simulink model "EvPowertrainController4EM"  (R2026b)
model workspace (MAT data in the model file):
  CtrlVcuAccelPdlBpts = [0 0.8 1]
  CtrlVcuBattPnlty = 10000000
  CtrlVcuBattSOCBpts = [0 20 60 80 100]
  CtrlVcuCnstrntPnltyFctr = 10000000
  CtrlVcuEMPnlty = 100
  CtrlVcuEMTrqSplitGrid = 200
  CtrlVcuFallRate = -500
  CtrlVcuMaxAccelG = 1
  CtrlVcuMaxDecelG = -1.5
  CtrlVcuPwrDeltaPnlty = 50
  CtrlVcuPwrRatePnlty = [25 25 100]
  CtrlVcuRiseRate = 500
  CtrlVcuRoadMuEst = 0.8
  CtrlVcuSftyFctr = 0.9
  CtrlVcuTracPwrErrPnlty = 25
  CtrlVcuTrqVecBrkThresh = 0.01
  CtrlVcuTrqVecIGain = 0
  CtrlVcuTrqVecMinTrq = 25
  CtrlVcuTrqVecPGain = -2000
  CtrlVcuTrqVecSteerThresh = 0.349065850399
  CtrlVcuTrqVecVelThresh = 2.5
  N_P0 = 3
undefined symbols (not defined in the file): CtrlBcuTrlrBrkGain, CtrlVcuEvChrgLmtBpt, CtrlVcuEvRegenBrkCutOff, CtrlVcuEvRegenBrkSpdBpt, CtrlVcuEvSocBpt, eff, EnvGrvty, PlntBrkActrBoreFrnt, PlntBrkActrBoreRear, PlntBrkFrntBias, PlntBrkKinFricCffFrnt, PlntBrkKinFricCffRear, PlntBrkNumPadsFrnt, PlntBrkNumPadsRear, PlntBrkPadMeanRadiusFrnt, PlntBrkPadMeanRadiusRear, PlntBrkPrsFctr, PlntBrkRearBias, PlntDiffrntl2Eff, PlntDiffrntl2Ratio, PlntDiffrntlEff, PlntDiffrntlRatio, PlntEM1EffTbl, PlntEM1Spd, PlntEM1SpdEff, PlntEM1TransEff, PlntEM1TransGearRatio, PlntEM1Trq, PlntEM1TrqEff, PlntEM2EffTbl, PlntEM2Spd, PlntEM2SpdEff, PlntEM2TransEff, PlntEM2TransGearRatio, PlntEM2Trq, PlntEM2TrqEff, PlntEM3EffTbl, PlntEM3Spd, PlntEM3SpdEff, PlntEM3TransEff, PlntEM3TransGearRatio, PlntEM3Trq, PlntEM3TrqEff, PlntEMWhlGearEffFL, PlntEMWhlGearEffRL, PlntEMWhlGearRatioFL, PlntEMWhlGearRatioRL, PlntTransEffSpdBpt, PlntTransEffTbl, PlntTransEffTempBpt, PlntTransEffTrqBpt, PlntTransGearNumVect, PlntTransGearRatioVect, PlntVehCGHgtAxl, PlntVehDstCGFrntAxl, PlntVehDstCGRearAxl, PlntVehMass, PlntWhlLdRadiusFrnt, PlntWhlLdRadiusRear
libraries: simulink x11, sl_discontinuities x6, autolibutils x2, slpidlib x2
(part 5 of 5)

== system EvPowertrainController4EM/Energy Management/Calculate Average EMSpd and Wheel Torque Curves for Front and Rear Axles/3EM Dual Front/EMTrq2WhlTrqFrnt/Single Speed Transmission/Gear Eta ==
  note: Pwr >= 0, v = 1
      | Pwr < 0, v= -1
  SpdIn : Inport
  TrqIn : Inport  Port=2
  Constant : Constant  Value=PlntEMWhlGearEffFL*PlntEM1TransEff
  Constant1 : Constant  SampleTime=-1
  Constant2 : Constant  Value=-1  SampleTime=-1
  Math Function1 : Math  Operator=pow  SignedPower=on  OutputSignalType=real
  Product1 : Product
  Switch2 : Switch  SaturateOnIntegerOverflow=off  InputSameDT=off
  eta : Outport  VectorParamsAs1DForOutWhenUnconnected=off
  wires:
  TrqIn/1 -> Product1/1
  Math Function1/1 -> eta/1
  Switch2/1 -> Math Function1/2
  Product1/1 -> Switch2/2
  Constant1/1 -> Switch2/1
  Constant2/1 -> Switch2/3
  Constant/1 -> Math Function1/1
  SpdIn/1 -> Product1/2

== system EvPowertrainController4EM/Energy Management/Calculate Average EMSpd and Wheel Torque Curves for Front and Rear Axles/3EM Dual Front/EMTrq2WhlTrqFrnt/Transmission/Diff Eta ==
  SpdIn : Inport
  TrqIn : Inport  Port=2
  Constant : Constant  Value=PlntDiffrntlEff
  Constant1 : Constant  SampleTime=-1
  Constant2 : Constant  Value=-1  SampleTime=-1
  Math Function1 : Math  Operator=pow  SignedPower=on  OutputSignalType=real
  Product1 : Product
  Switch2 : Switch  SaturateOnIntegerOverflow=off  InputSameDT=off
  eta : Outport  VectorParamsAs1DForOutWhenUnconnected=off
  wires:
  TrqIn/1 -> Product1/1
  Math Function1/1 -> eta/1
  Switch2/1 -> Math Function1/2
  Product1/1 -> Switch2/2
  Constant1/1 -> Switch2/1
  Constant2/1 -> Switch2/3
  Constant/1 -> Math Function1/1
  SpdIn/1 -> Product1/2

== system EvPowertrainController4EM/Energy Management/Calculate Average EMSpd and Wheel Torque Curves for Front and Rear Axles/3EM Dual Front/EMTrq2WhlTrqFrnt/Transmission/Trans Eta ==
  TrqIn : Inport
  SpdIn : Inport  Port=2
  Gear : Inport  Port=3
  Abs1 : Abs  SaturateOnIntegerOverflow=off
  Constant : Constant  Value=PlntTransEffTempBpt(1)
  Constant1 : Constant  SampleTime=-1
  Constant2 : Constant  Value=-1  SampleTime=-1
  Eta 4D : Lookup_n-D  NumberOfTableDimensions=4  LookupTableObject=''  BreakpointsForDimension1=PlntTransEffTrqBpt  BreakpointsForDimension2=PlntTransEffSpdBpt  BreakpointsForDimension3=PlntTransGearNumVect  BreakpointsForDimension4=PlntTransEffTempBpt  Table=PlntTransEffTbl  ExtrapMethod=Clip  InternalRulePriority=Speed  RndMeth=Simplest
      settings: InputPortMap=u0,u1,u2,u3
  Math Function1 : Math  Operator=pow  SignedPower=on  OutputSignalType=real
  Product1 : Product
  Switch2 : Switch  SaturateOnIntegerOverflow=off  InputSameDT=off
  eta : Outport  VectorParamsAs1DForOutWhenUnconnected=off
  wires:
  Constant/1 -> Eta 4D/4
  Gear/1 -> Eta 4D/3
  SpdIn/1 -> Eta 4D/2, Product1/2
  Eta 4D/1 -> Math Function1/1
  Constant2/1 -> Switch2/3
  Constant1/1 -> Switch2/1
  Product1/1 -> Switch2/2
  Switch2/1 -> Math Function1/2
  Abs1/1 -> Eta 4D/1
  Math Function1/1 -> eta/1
  TrqIn/1 -> Abs1/1, Product1/1

== system EvPowertrainController4EM/Energy Management/Calculate Average EMSpd and Wheel Torque Curves for Front and Rear Axles/3EM Dual Front/EMTrq2WhlTrqRear/Single Speed Transmission/Diff Eta ==
  note: Pwr >= 0, v = 1
      | Pwr < 0, v= -1
  SpdIn : Inport
  TrqIn : Inport  Port=2
  Constant : Constant  Value=PlntDiffrntl2Eff*PlntEM3TransEff
  Constant1 : Constant  SampleTime=-1
  Constant2 : Constant  Value=-1  SampleTime=-1
  Math Function1 : Math  Operator=pow  SignedPower=on  OutputSignalType=real
  Product1 : Product
  Switch2 : Switch  SaturateOnIntegerOverflow=off  InputSameDT=off
  eta : Outport  VectorParamsAs1DForOutWhenUnconnected=off
  wires:
  TrqIn/1 -> Product1/1
  Math Function1/1 -> eta/1
  Switch2/1 -> Math Function1/2
  Product1/1 -> Switch2/2
  Constant1/1 -> Switch2/1
  Constant2/1 -> Switch2/3
  Constant/1 -> Math Function1/1
  SpdIn/1 -> Product1/2

== system EvPowertrainController4EM/Energy Management/Calculate Average EMSpd and Wheel Torque Curves for Front and Rear Axles/3EM Dual Front/EMTrq2WhlTrqRear/Transmission/Diff Eta ==
  SpdIn : Inport
  TrqIn : Inport  Port=2
  Constant : Constant  Value=PlntDiffrntl2Eff
  Constant1 : Constant  SampleTime=-1
  Constant2 : Constant  Value=-1  SampleTime=-1
  Math Function1 : Math  Operator=pow  SignedPower=on  OutputSignalType=real
  Product1 : Product
  Switch2 : Switch  SaturateOnIntegerOverflow=off  InputSameDT=off
  eta : Outport  VectorParamsAs1DForOutWhenUnconnected=off
  wires:
  SpdIn/1 -> Product1/2
  Constant/1 -> Math Function1/1
  Constant2/1 -> Switch2/3
  Constant1/1 -> Switch2/1
  Product1/1 -> Switch2/2
  Switch2/1 -> Math Function1/2
  Math Function1/1 -> eta/1
  TrqIn/1 -> Product1/1

== system EvPowertrainController4EM/Energy Management/Calculate Average EMSpd and Wheel Torque Curves for Front and Rear Axles/3EM Dual Front/EMTrq2WhlTrqRear/Transmission/Trans Eta ==
  TrqIn : Inport
  SpdIn : Inport  Port=2
  Gear : Inport  Port=3
  Abs1 : Abs  SaturateOnIntegerOverflow=off
  Constant : Constant  Value=PlntTransEffTempBpt(1)
  Constant1 : Constant  SampleTime=-1
  Constant2 : Constant  Value=-1  SampleTime=-1
  Eta 4D : Lookup_n-D  NumberOfTableDimensions=4  LookupTableObject=''  BreakpointsForDimension1=PlntTransEffTrqBpt  BreakpointsForDimension2=PlntTransEffSpdBpt  BreakpointsForDimension3=PlntTransGearNumVect  BreakpointsForDimension4=PlntTransEffTempBpt  Table=PlntTransEffTbl  ExtrapMethod=Clip  InternalRulePriority=Speed  RndMeth=Simplest
      settings: InputPortMap=u0,u1,u2,u3
  Math Function1 : Math  Operator=pow  SignedPower=on  OutputSignalType=real
  Product1 : Product
  Switch2 : Switch  SaturateOnIntegerOverflow=off  InputSameDT=off
  eta : Outport  VectorParamsAs1DForOutWhenUnconnected=off
  wires:
  TrqIn/1 -> Product1/1, Abs1/1
  Math Function1/1 -> eta/1
  Abs1/1 -> Eta 4D/1
  Switch2/1 -> Math Function1/2
  Product1/1 -> Switch2/2
  Constant1/1 -> Switch2/1
  Constant2/1 -> Switch2/3
  Eta 4D/1 -> Math Function1/1
  SpdIn/1 -> Product1/2, Eta 4D/2
  Gear/1 -> Eta 4D/3
  Constant/1 -> Eta 4D/4

== system EvPowertrainController4EM/Energy Management/Calculate Average EMSpd and Wheel Torque Curves for Front and Rear Axles/3EM Dual Rear/EMTrq2WhlTrqFrnt/Single Speed Transmission/Diff Eta ==
  note: Pwr >= 0, v = 1
      | Pwr < 0, v= -1
  SpdIn : Inport
  TrqIn : Inport  Port=2
  Constant : Constant  Value=PlntDiffrntlEff*PlntEM1TransEff
  Constant1 : Constant  SampleTime=-1
  Constant2 : Constant  Value=-1  SampleTime=-1
  Math Function1 : Math  Operator=pow  SignedPower=on  OutputSignalType=real
  Product1 : Product
  Switch2 : Switch  SaturateOnIntegerOverflow=off  InputSameDT=off
  eta : Outport  VectorParamsAs1DForOutWhenUnconnected=off
  wires:
  SpdIn/1 -> Product1/2
  Constant/1 -> Math Function1/1
  Constant2/1 -> Switch2/3
  Constant1/1 -> Switch2/1
  Product1/1 -> Switch2/2
  Switch2/1 -> Math Function1/2
  Math Function1/1 -> eta/1
  TrqIn/1 -> Product1/1

== system EvPowertrainController4EM/Energy Management/Calculate Average EMSpd and Wheel Torque Curves for Front and Rear Axles/3EM Dual Rear/EMTrq2WhlTrqFrnt/Transmission/Diff Eta ==
  SpdIn : Inport
  TrqIn : Inport  Port=2
  Constant : Constant  Value=PlntDiffrntlEff
  Constant1 : Constant  SampleTime=-1
  Constant2 : Constant  Value=-1  SampleTime=-1
  Math Function1 : Math  Operator=pow  SignedPower=on  OutputSignalType=real
  Product1 : Product
  Switch2 : Switch  SaturateOnIntegerOverflow=off  InputSameDT=off
  eta : Outport  VectorParamsAs1DForOutWhenUnconnected=off
  wires:
  SpdIn/1 -> Product1/2
  Constant/1 -> Math Function1/1
  Constant2/1 -> Switch2/3
  Constant1/1 -> Switch2/1
  Product1/1 -> Switch2/2
  Switch2/1 -> Math Function1/2
  Math Function1/1 -> eta/1
  TrqIn/1 -> Product1/1

== system EvPowertrainController4EM/Energy Management/Calculate Average EMSpd and Wheel Torque Curves for Front and Rear Axles/3EM Dual Rear/EMTrq2WhlTrqFrnt/Transmission/Trans Eta ==
  TrqIn : Inport
  SpdIn : Inport  Port=2
  Gear : Inport  Port=3
  Abs1 : Abs  SaturateOnIntegerOverflow=off
  Constant : Constant  Value=PlntTransEffTempBpt(1)
  Constant1 : Constant  SampleTime=-1
  Constant2 : Constant  Value=-1  SampleTime=-1
  Eta 4D : Lookup_n-D  NumberOfTableDimensions=4  LookupTableObject=''  BreakpointsForDimension1=PlntTransEffTrqBpt  BreakpointsForDimension2=PlntTransEffSpdBpt  BreakpointsForDimension3=PlntTransGearNumVect  BreakpointsForDimension4=PlntTransEffTempBpt  Table=PlntTransEffTbl  ExtrapMethod=Clip  InternalRulePriority=Speed  RndMeth=Simplest
      settings: InputPortMap=u0,u1,u2,u3
  Math Function1 : Math  Operator=pow  SignedPower=on  OutputSignalType=real
  Product1 : Product
  Switch2 : Switch  SaturateOnIntegerOverflow=off  InputSameDT=off
  eta : Outport  VectorParamsAs1DForOutWhenUnconnected=off
  wires:
  TrqIn/1 -> Product1/1, Abs1/1
  Math Function1/1 -> eta/1
  Abs1/1 -> Eta 4D/1
  Switch2/1 -> Math Function1/2
  Product1/1 -> Switch2/2
  Constant1/1 -> Switch2/1
  Constant2/1 -> Switch2/3
  Eta 4D/1 -> Math Function1/1
  SpdIn/1 -> Product1/2, Eta 4D/2
  Gear/1 -> Eta 4D/3
  Constant/1 -> Eta 4D/4

== system EvPowertrainController4EM/Energy Management/Calculate Average EMSpd and Wheel Torque Curves for Front and Rear Axles/3EM Dual Rear/EMTrq2WhlTrqRear/Single Speed Transmission/Gear Eta ==
  note: Pwr >= 0, v = 1
      | Pwr < 0, v= -1
  SpdIn : Inport
  TrqIn : Inport  Port=2
  Constant : Constant  Value=PlntEMWhlGearEffRL*PlntEM2TransEff
  Constant1 : Constant  SampleTime=-1
  Constant2 : Constant  Value=-1  SampleTime=-1
  Math Function1 : Math  Operator=pow  SignedPower=on  OutputSignalType=real
  Product1 : Product
  Switch2 : Switch  SaturateOnIntegerOverflow=off  InputSameDT=off
  eta : Outport  VectorParamsAs1DForOutWhenUnconnected=off
  wires:
  SpdIn/1 -> Product1/2
  Constant/1 -> Math Function1/1
  Constant2/1 -> Switch2/3
  Constant1/1 -> Switch2/1
  Product1/1 -> Switch2/2
  Switch2/1 -> Math Function1/2
  Math Function1/1 -> eta/1
  TrqIn/1 -> Product1/1

== system EvPowertrainController4EM/Energy Management/Calculate Average EMSpd and Wheel Torque Curves for Front and Rear Axles/3EM Dual Rear/EMTrq2WhlTrqRear/Transmission/Diff Eta ==
  SpdIn : Inport
  TrqIn : Inport  Port=2
  Constant : Constant  Value=PlntDiffrntl2Eff
  Constant1 : Constant  SampleTime=-1
  Constant2 : Constant  Value=-1  SampleTime=-1
  Math Function1 : Math  Operator=pow  SignedPower=on  OutputSignalType=real
  Product1 : Product
  Switch2 : Switch  SaturateOnIntegerOverflow=off  InputSameDT=off
  eta : Outport  VectorParamsAs1DForOutWhenUnconnected=off
  wires:
  TrqIn/1 -> Product1/1
  Math Function1/1 -> eta/1
  Switch2/1 -> Math Function1/2
  Product1/1 -> Switch2/2
  Constant1/1 -> Switch2/1
  Constant2/1 -> Switch2/3
  Constant/1 -> Math Function1/1
  SpdIn/1 -> Product1/2

== system EvPowertrainController4EM/Energy Management/Calculate Average EMSpd and Wheel Torque Curves for Front and Rear Axles/3EM Dual Rear/EMTrq2WhlTrqRear/Transmission/Trans Eta ==
  TrqIn : Inport
  SpdIn : Inport  Port=2
  Gear : Inport  Port=3
  Abs1 : Abs  SaturateOnIntegerOverflow=off
  Constant : Constant  Value=PlntTransEffTempBpt(1)
  Constant1 : Constant  SampleTime=-1
  Constant2 : Constant  Value=-1  SampleTime=-1
  Eta 4D : Lookup_n-D  NumberOfTableDimensions=4  LookupTableObject=''  BreakpointsForDimension1=PlntTransEffTrqBpt  BreakpointsForDimension2=PlntTransEffSpdBpt  BreakpointsForDimension3=PlntTransGearNumVect  BreakpointsForDimension4=PlntTransEffTempBpt  Table=PlntTransEffTbl  ExtrapMethod=Clip  InternalRulePriority=Speed  RndMeth=Simplest
      settings: InputPortMap=u0,u1,u2,u3
  Math Function1 : Math  Operator=pow  SignedPower=on  OutputSignalType=real
  Product1 : Product
  Switch2 : Switch  SaturateOnIntegerOverflow=off  InputSameDT=off
  eta : Outport  VectorParamsAs1DForOutWhenUnconnected=off
  wires:
  Constant/1 -> Eta 4D/4
  Gear/1 -> Eta 4D/3
  SpdIn/1 -> Eta 4D/2, Product1/2
  Eta 4D/1 -> Math Function1/1
  Constant2/1 -> Switch2/3
  Constant1/1 -> Switch2/1
  Product1/1 -> Switch2/2
  Switch2/1 -> Math Function1/2
  Abs1/1 -> Eta 4D/1
  Math Function1/1 -> eta/1
  TrqIn/1 -> Abs1/1, Product1/1

== system EvPowertrainController4EM/Energy Management/Calculate Average EMSpd and Wheel Torque Curves for Front and Rear Axles/4EM/EMTrq2WhlTrqFrnt/Single Speed Transmission/Gear Eta ==
  SpdIn : Inport
  TrqIn : Inport  Port=2
  Constant : Constant  Value=PlntEMWhlGearEffFL*PlntEM1TransEff
  Constant1 : Constant  SampleTime=-1
  Constant2 : Constant  Value=-1  SampleTime=-1
  Math Function1 : Math  Operator=pow  SignedPower=on  OutputSignalType=real
  Product1 : Product
  Switch2 : Switch  SaturateOnIntegerOverflow=off  InputSameDT=off
  eta : Outport  VectorParamsAs1DForOutWhenUnconnected=off
  wires:
  TrqIn/1 -> Product1/1
  Math Function1/1 -> eta/1
  Switch2/1 -> Math Function1/2
  Product1/1 -> Switch2/2
  Constant1/1 -> Switch2/1
  Constant2/1 -> Switch2/3
  Constant/1 -> Math Function1/1
  SpdIn/1 -> Product1/2

== system EvPowertrainController4EM/Energy Management/Calculate Average EMSpd and Wheel Torque Curves for Front and Rear Axles/4EM/EMTrq2WhlTrqFrnt/Transmission/Diff Eta ==
  SpdIn : Inport
  TrqIn : Inport  Port=2
  Constant : Constant  Value=PlntDiffrntlEff
  Constant1 : Constant  SampleTime=-1
  Constant2 : Constant  Value=-1  SampleTime=-1
  Math Function1 : Math  Operator=pow  SignedPower=on  OutputSignalType=real
  Product1 : Product
  Switch2 : Switch  SaturateOnIntegerOverflow=off  InputSameDT=off
  eta : Outport  VectorParamsAs1DForOutWhenUnconnected=off
  wires:
  TrqIn/1 -> Product1/1
  Math Function1/1 -> eta/1
  Switch2/1 -> Math Function1/2
  Product1/1 -> Switch2/2
  Constant1/1 -> Switch2/1
  Constant2/1 -> Switch2/3
  Constant/1 -> Math Function1/1
  SpdIn/1 -> Product1/2

== system EvPowertrainController4EM/Energy Management/Calculate Average EMSpd and Wheel Torque Curves for Front and Rear Axles/4EM/EMTrq2WhlTrqFrnt/Transmission/Trans Eta ==
  TrqIn : Inport
  SpdIn : Inport  Port=2
  Gear : Inport  Port=3
  Abs1 : Abs  SaturateOnIntegerOverflow=off
  Constant : Constant  Value=PlntTransEffTempBpt(1)
  Constant1 : Constant  SampleTime=-1
  Constant2 : Constant  Value=-1  SampleTime=-1
  Eta 4D : Lookup_n-D  NumberOfTableDimensions=4  LookupTableObject=''  BreakpointsForDimension1=PlntTransEffTrqBpt  BreakpointsForDimension2=PlntTransEffSpdBpt  BreakpointsForDimension3=PlntTransGearNumVect  BreakpointsForDimension4=PlntTransEffTempBpt  Table=PlntTransEffTbl  ExtrapMethod=Clip  InternalRulePriority=Speed  RndMeth=Simplest
      settings: InputPortMap=u0,u1,u2,u3
  Math Function1 : Math  Operator=pow  SignedPower=on  OutputSignalType=real
  Product1 : Product
  Switch2 : Switch  SaturateOnIntegerOverflow=off  InputSameDT=off
  eta : Outport  VectorParamsAs1DForOutWhenUnconnected=off
  wires:
  Constant/1 -> Eta 4D/4
  Gear/1 -> Eta 4D/3
  SpdIn/1 -> Eta 4D/2, Product1/2
  Eta 4D/1 -> Math Function1/1
  Constant2/1 -> Switch2/3
  Constant1/1 -> Switch2/1
  Product1/1 -> Switch2/2
  Switch2/1 -> Math Function1/2
  Abs1/1 -> Eta 4D/1
  Math Function1/1 -> eta/1
  TrqIn/1 -> Abs1/1, Product1/1

== system EvPowertrainController4EM/Energy Management/Calculate Average EMSpd and Wheel Torque Curves for Front and Rear Axles/4EM/EMTrq2WhlTrqRear/Single Speed Transmission/Gear Eta ==
  SpdIn : Inport
  TrqIn : Inport  Port=2
  Constant : Constant  Value=PlntEMWhlGearEffRL*PlntEM3TransEff
  Constant1 : Constant  SampleTime=-1
  Constant2 : Constant  Value=-1  SampleTime=-1
  Math Function1 : Math  Operator=pow  SignedPower=on  OutputSignalType=real
  Product1 : Product
  Switch2 : Switch  SaturateOnIntegerOverflow=off  InputSameDT=off
  eta : Outport  VectorParamsAs1DForOutWhenUnconnected=off
  wires:
  TrqIn/1 -> Product1/1
  Math Function1/1 -> eta/1
  Switch2/1 -> Math Function1/2
  Product1/1 -> Switch2/2
  Constant1/1 -> Switch2/1
  Constant2/1 -> Switch2/3
  Constant/1 -> Math Function1/1
  SpdIn/1 -> Product1/2

== system EvPowertrainController4EM/Energy Management/Calculate Average EMSpd and Wheel Torque Curves for Front and Rear Axles/4EM/EMTrq2WhlTrqRear/Transmission/Diff Eta ==
  SpdIn : Inport
  TrqIn : Inport  Port=2
  Constant : Constant  Value=PlntDiffrntl2Eff
  Constant1 : Constant  SampleTime=-1
  Constant2 : Constant  Value=-1  SampleTime=-1
  Math Function1 : Math  Operator=pow  SignedPower=on  OutputSignalType=real
  Product1 : Product
  Switch2 : Switch  SaturateOnIntegerOverflow=off  InputSameDT=off
  eta : Outport  VectorParamsAs1DForOutWhenUnconnected=off
  wires:
  SpdIn/1 -> Product1/2
  Constant/1 -> Math Function1/1
  Constant2/1 -> Switch2/3
  Constant1/1 -> Switch2/1
  Product1/1 -> Switch2/2
  Switch2/1 -> Math Function1/2
  Math Function1/1 -> eta/1
  TrqIn/1 -> Product1/1

== system EvPowertrainController4EM/Energy Management/Calculate Average EMSpd and Wheel Torque Curves for Front and Rear Axles/4EM/EMTrq2WhlTrqRear/Transmission/Trans Eta ==
  TrqIn : Inport
  SpdIn : Inport  Port=2
  Gear : Inport  Port=3
  Abs1 : Abs  SaturateOnIntegerOverflow=off
  Constant : Constant  Value=PlntTransEffTempBpt(1)
  Constant1 : Constant  SampleTime=-1
  Constant2 : Constant  Value=-1  SampleTime=-1
  Eta 4D : Lookup_n-D  NumberOfTableDimensions=4  LookupTableObject=''  BreakpointsForDimension1=PlntTransEffTrqBpt  BreakpointsForDimension2=PlntTransEffSpdBpt  BreakpointsForDimension3=PlntTransGearNumVect  BreakpointsForDimension4=PlntTransEffTempBpt  Table=PlntTransEffTbl  ExtrapMethod=Clip  InternalRulePriority=Speed  RndMeth=Simplest
      settings: InputPortMap=u0,u1,u2,u3
  Math Function1 : Math  Operator=pow  SignedPower=on  OutputSignalType=real
  Product1 : Product
  Switch2 : Switch  SaturateOnIntegerOverflow=off  InputSameDT=off
  eta : Outport  VectorParamsAs1DForOutWhenUnconnected=off
  wires:
  TrqIn/1 -> Product1/1, Abs1/1
  Math Function1/1 -> eta/1
  Abs1/1 -> Eta 4D/1
  Switch2/1 -> Math Function1/2
  Product1/1 -> Switch2/2
  Constant1/1 -> Switch2/1
  Constant2/1 -> Switch2/3
  Eta 4D/1 -> Math Function1/1
  SpdIn/1 -> Product1/2, Eta 4D/2
  Gear/1 -> Eta 4D/3
  Constant/1 -> Eta 4D/4

== system EvPowertrainController4EM/Energy Management/Powertrain Constraints /Battery Constraint/Electrical Current/DC-DC Eta/DC-DC Eta ==
  In : Inport
  DCDC Constant Eff : Gain  Gain=1+(100-eff)/100
  Out : Outport  VectorParamsAs1DForOutWhenUnconnected=off
  wires:
  DCDC Constant Eff/1 -> Out/1
  In/1 -> DCDC Constant Eff/1

== system EvPowertrainController4EM/Energy Management/Powertrain Constraints /Battery Constraint/Electrical Current/DC-DC Eta/No DC-DC ==
  In : Inport
  Out : Outport  VectorParamsAs1DForOutWhenUnconnected=off
  wires:
  In/1 -> Out/1

== system EvPowertrainController4EM/Energy Management/Powertrain Constraints /EM Constraint Front/Tabular Power Loss Data/2EM or 3EM Dual Rear/WhlTrq2EMTrq ==
  EMSpd : Inport
  WhlTrqCmd : Inport  Port=2
  Diff Eta : Subsystem
  Divide2 : Product  Inputs=/*
  Gain3 : Gain  Gain=1/(PlntDiffrntlRatio*PlntEM1TransGearRatio)
  Unit Delay : UnitDelay  SampleTime=-1
  EMTrq : Outport  VectorParamsAs1DForOutWhenUnconnected=off
  wires:
  Unit Delay/1 -> Diff Eta/2(TrqIn)
  Diff Eta/1(eta) -> Divide2/1
  WhlTrqCmd/1 -> Gain3/1
  EMSpd/1 -> Diff Eta/1(SpdIn)
  Divide2/1 -> EMTrq/1, Unit Delay/1
  Gain3/1 -> Divide2/2

== system EvPowertrainController4EM/Energy Management/Powertrain Constraints /EM Constraint Front/Tabular Power Loss Data/3EM Dual Front or 4EM/WhlTrq2EMTrq ==
  EMSpd : Inport
  WhlTrqCmd : Inport  Port=2
  Divide2 : Product  Inputs=/*
  Dual EMs : Gain  Gain=1/2
  Gain3 : Gain  Gain=1/(PlntEMWhlGearRatioFL*PlntEM1TransGearRatio)
  Gear Eta : Subsystem
  Unit Delay : UnitDelay  SampleTime=-1
  EMTrq : Outport  VectorParamsAs1DForOutWhenUnconnected=off
  wires:
  Dual EMs/1 -> Gain3/1
  Gain3/1 -> Divide2/2
  Divide2/1 -> Unit Delay/1, EMTrq/1
  EMSpd/1 -> Gear Eta/1(SpdIn)
  WhlTrqCmd/1 -> Dual EMs/1
  Gear Eta/1(eta) -> Divide2/1
  Unit Delay/1 -> Gear Eta/2(TrqIn)

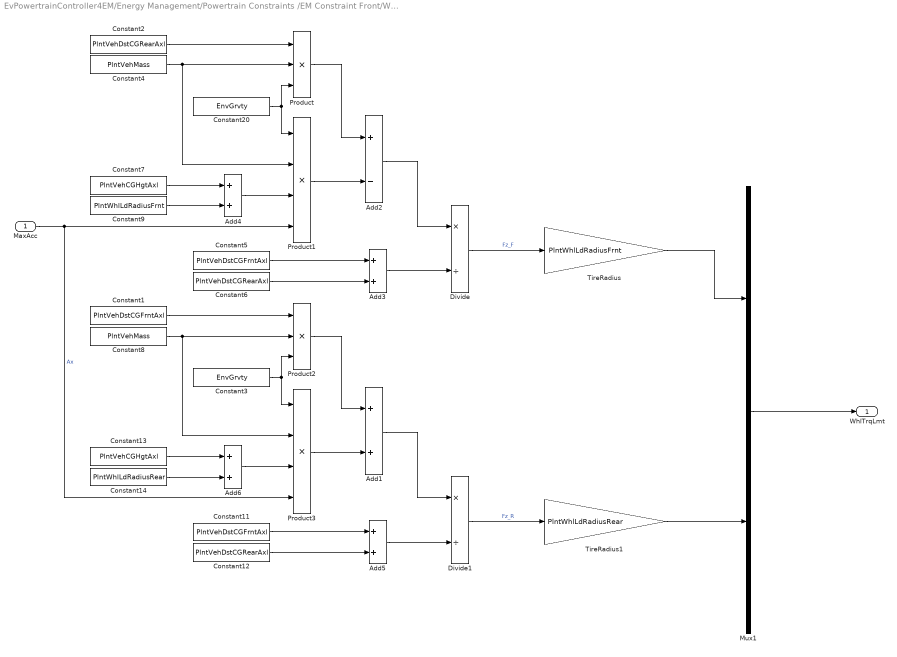
== system EvPowertrainController4EM/Energy Management/Powertrain Constraints /EM Constraint Front/Wheel Torque Saturation for Max g Rates/Wheel Torque Limit at Max g Rates/Wheel Torque at Max Acceleration Rate ==
  MaxAcc : Inport
  Add{1,3..6} (5 alike) : Sum
  Add2 : Sum  Inputs=+-
  Constant1 : Constant  Value=PlntVehDstCGFrntAxl  SampleTime=-1
  Constant11 : Constant  Value=PlntVehDstCGFrntAxl  SampleTime=-1
  Constant12 : Constant  Value=PlntVehDstCGRearAxl  SampleTime=-1
  Constant13 : Constant  Value=PlntVehCGHgtAxl  SampleTime=-1
  Constant14 : Constant  Value=PlntWhlLdRadiusRear  SampleTime=-1
  Constant2 : Constant  Value=PlntVehDstCGRearAxl  SampleTime=-1
  Constant20 : Constant  Value=EnvGrvty  SampleTime=-1
  Constant3 : Constant  Value=EnvGrvty  SampleTime=-1
  Constant4 : Constant  Value=PlntVehMass  SampleTime=-1
  Constant5 : Constant  Value=PlntVehDstCGFrntAxl  SampleTime=-1
  Constant6 : Constant  Value=PlntVehDstCGRearAxl  SampleTime=-1
  Constant7 : Constant  Value=PlntVehCGHgtAxl  SampleTime=-1
  Constant8 : Constant  Value=PlntVehMass  SampleTime=-1
  Constant9 : Constant  Value=PlntWhlLdRadiusFrnt  SampleTime=-1
  Divide : Product  Inputs=*/
  Divide1 : Product  Inputs=*/
  Mux1 : Mux  Inputs=2
  Product : Product  Inputs=3
  Product1 : Product  Inputs=4
  Product2 : Product  Inputs=3
  Product3 : Product  Inputs=4
  TireRadius : Gain  Gain=PlntWhlLdRadiusFrnt
  TireRadius1 : Gain  Gain=PlntWhlLdRadiusRear
  WhlTrqLmt : Outport  VectorParamsAs1DForOutWhenUnconnected=off
  wires:
  Divide1/1 -> TireRadius1/1  "Fz_R"
  Product3/1 -> Add1/2
  Product2/1 -> Add1/1
  Constant11/1 -> Add5/1
  Constant8/1 -> Product3/2, Product2/2
  Add5/1 -> Divide1/2
  Add6/1 -> Product3/3
  Constant12/1 -> Add5/2
  Constant1/1 -> Product2/1
  Constant13/1 -> Add6/1
  Constant14/1 -> Add6/2
  Add1/1 -> Divide1/1
  Constant3/1 -> Product3/1, Product2/3
  Constant20/1 -> Product/3, Product1/1
  Mux1/1 -> WhlTrqLmt/1
  Add2/1 -> Divide/1
  Constant9/1 -> Add4/2
  Constant7/1 -> Add4/1
  Constant2/1 -> Product/1
  Constant6/1 -> Add3/2
  Divide/1 -> TireRadius/1  "Fz_F"
  Add4/1 -> Product1/3
  Add3/1 -> Divide/2
  MaxAcc/1 -> Product1/4, Product3/4  "Ax"
  Constant4/1 -> Product/2, Product1/2
  Constant5/1 -> Add3/1
  Product/1 -> Add2/1
  Product1/1 -> Add2/2
  TireRadius/1 -> Mux1/1
  TireRadius1/1 -> Mux1/2

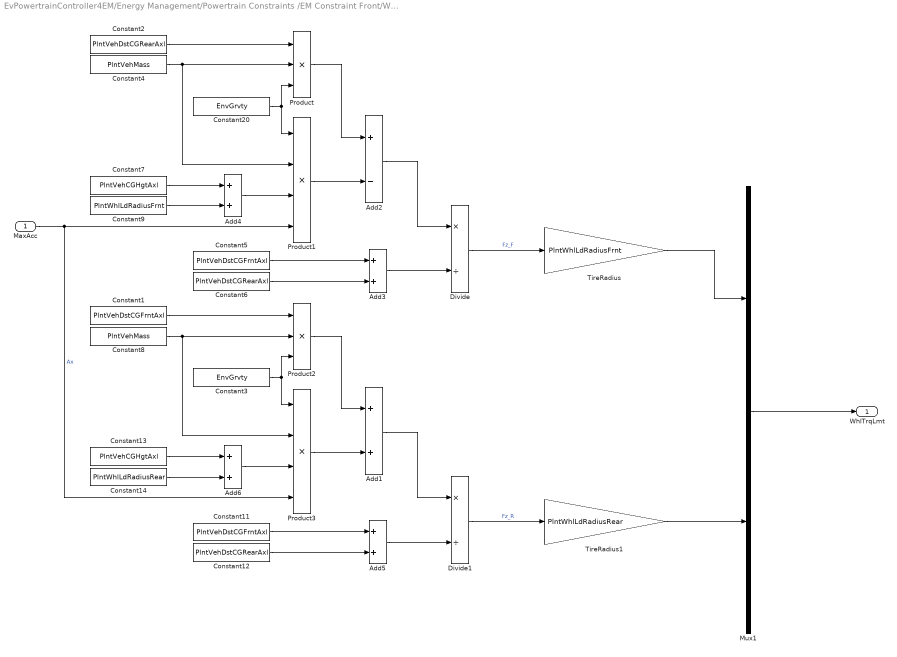
== system EvPowertrainController4EM/Energy Management/Powertrain Constraints /EM Constraint Front/Wheel Torque Saturation for Max g Rates/Wheel Torque Limit at Max g Rates/Wheel Torque at Max Deceleration Rate ==
  MaxAcc : Inport
  Add{1,3..6} (5 alike) : Sum
  Add2 : Sum  Inputs=+-
  Constant1 : Constant  Value=PlntVehDstCGFrntAxl  SampleTime=-1
  Constant11 : Constant  Value=PlntVehDstCGFrntAxl  SampleTime=-1
  Constant12 : Constant  Value=PlntVehDstCGRearAxl  SampleTime=-1
  Constant13 : Constant  Value=PlntVehCGHgtAxl  SampleTime=-1
  Constant14 : Constant  Value=PlntWhlLdRadiusRear  SampleTime=-1
  Constant2 : Constant  Value=PlntVehDstCGRearAxl  SampleTime=-1
  Constant20 : Constant  Value=EnvGrvty  SampleTime=-1
  Constant3 : Constant  Value=EnvGrvty  SampleTime=-1
  Constant4 : Constant  Value=PlntVehMass  SampleTime=-1
  Constant5 : Constant  Value=PlntVehDstCGFrntAxl  SampleTime=-1
  Constant6 : Constant  Value=PlntVehDstCGRearAxl  SampleTime=-1
  Constant7 : Constant  Value=PlntVehCGHgtAxl  SampleTime=-1
  Constant8 : Constant  Value=PlntVehMass  SampleTime=-1
  Constant9 : Constant  Value=PlntWhlLdRadiusFrnt  SampleTime=-1
  Divide : Product  Inputs=*/
  Divide1 : Product  Inputs=*/
  Mux1 : Mux  Inputs=2
  Product : Product  Inputs=3
  Product1 : Product  Inputs=4
  Product2 : Product  Inputs=3
  Product3 : Product  Inputs=4
  TireRadius : Gain  Gain=PlntWhlLdRadiusFrnt
  TireRadius1 : Gain  Gain=PlntWhlLdRadiusRear
  WhlTrqLmt : Outport  VectorParamsAs1DForOutWhenUnconnected=off
  wires:
  TireRadius1/1 -> Mux1/2
  TireRadius/1 -> Mux1/1
  Product1/1 -> Add2/2
  Product/1 -> Add2/1
  Constant5/1 -> Add3/1
  Constant4/1 -> Product1/2, Product/2
  MaxAcc/1 -> Product3/4, Product1/4  "Ax"
  Add3/1 -> Divide/2
  Add4/1 -> Product1/3
  Divide/1 -> TireRadius/1  "Fz_F"
  Constant6/1 -> Add3/2
  Constant2/1 -> Product/1
  Constant7/1 -> Add4/1
  Constant9/1 -> Add4/2
  Add2/1 -> Divide/1
  Mux1/1 -> WhlTrqLmt/1
  Constant20/1 -> Product1/1, Product/3
  Constant3/1 -> Product2/3, Product3/1
  Add1/1 -> Divide1/1
  Constant14/1 -> Add6/2
  Constant13/1 -> Add6/1
  Constant1/1 -> Product2/1
  Constant12/1 -> Add5/2
  Add6/1 -> Product3/3
  Add5/1 -> Divide1/2
  Constant8/1 -> Product2/2, Product3/2
  Constant11/1 -> Add5/1
  Product2/1 -> Add1/1
  Product3/1 -> Add1/2
  Divide1/1 -> TireRadius1/1  "Fz_R"

== system EvPowertrainController4EM/Energy Management/Powertrain Constraints /EM Constraint Rear/Tabular Power Loss Data/2EM/WhlTrq2EMTrq ==
  EMSpd : Inport
  WhlTrqCmd : Inport  Port=2
  Diff Eta : Subsystem
  Divide2 : Product  Inputs=/*
  Gain3 : Gain  Gain=1/(PlntDiffrntl2Ratio*PlntEM2TransGearRatio)
  Unit Delay : UnitDelay  SampleTime=-1
  EMTrq : Outport  VectorParamsAs1DForOutWhenUnconnected=off
  wires:
  Unit Delay/1 -> Diff Eta/2(TrqIn)
  Diff Eta/1(eta) -> Divide2/1
  WhlTrqCmd/1 -> Gain3/1
  EMSpd/1 -> Diff Eta/1(SpdIn)
  Divide2/1 -> EMTrq/1, Unit Delay/1
  Gain3/1 -> Divide2/2

== system EvPowertrainController4EM/Energy Management/Powertrain Constraints /EM Constraint Rear/Tabular Power Loss Data/3EM Dual Front/WhlTrq2EMTrq ==
  EMSpd : Inport
  WhlTrqCmd : Inport  Port=2
  Diff Eta : Subsystem
  Divide2 : Product  Inputs=/*
  Gain3 : Gain  Gain=1/(PlntDiffrntl2Ratio*PlntEM3TransGearRatio)
  Unit Delay : UnitDelay  SampleTime=-1
  EMTrq : Outport  VectorParamsAs1DForOutWhenUnconnected=off
  wires:
  Gain3/1 -> Divide2/2
  Divide2/1 -> Unit Delay/1, EMTrq/1
  EMSpd/1 -> Diff Eta/1(SpdIn)
  WhlTrqCmd/1 -> Gain3/1
  Diff Eta/1(eta) -> Divide2/1
  Unit Delay/1 -> Diff Eta/2(TrqIn)

== system EvPowertrainController4EM/Energy Management/Powertrain Constraints /EM Constraint Rear/Tabular Power Loss Data/3EM Dual Rear or 4EM/WhlTrq2EMTrq ==
  EMSpd : Inport
  WhlTrqCmd : Inport  Port=2
  Divide2 : Product  Inputs=/*
  Dual EMs : Gain  Gain=1/2
  Gain3 : Gain  Gain=1/(PlntEMWhlGearRatioRL*PlntEM3TransGearRatio)
  Gear Eta : Subsystem
  Unit Delay : UnitDelay  SampleTime=-1
  EMTrq : Outport  VectorParamsAs1DForOutWhenUnconnected=off
  wires:
  Dual EMs/1 -> Gain3/1
  Gain3/1 -> Divide2/2
  Divide2/1 -> Unit Delay/1, EMTrq/1
  EMSpd/1 -> Gear Eta/1(SpdIn)
  WhlTrqCmd/1 -> Dual EMs/1
  Gear Eta/1(eta) -> Divide2/1
  Unit Delay/1 -> Gear Eta/2(TrqIn)

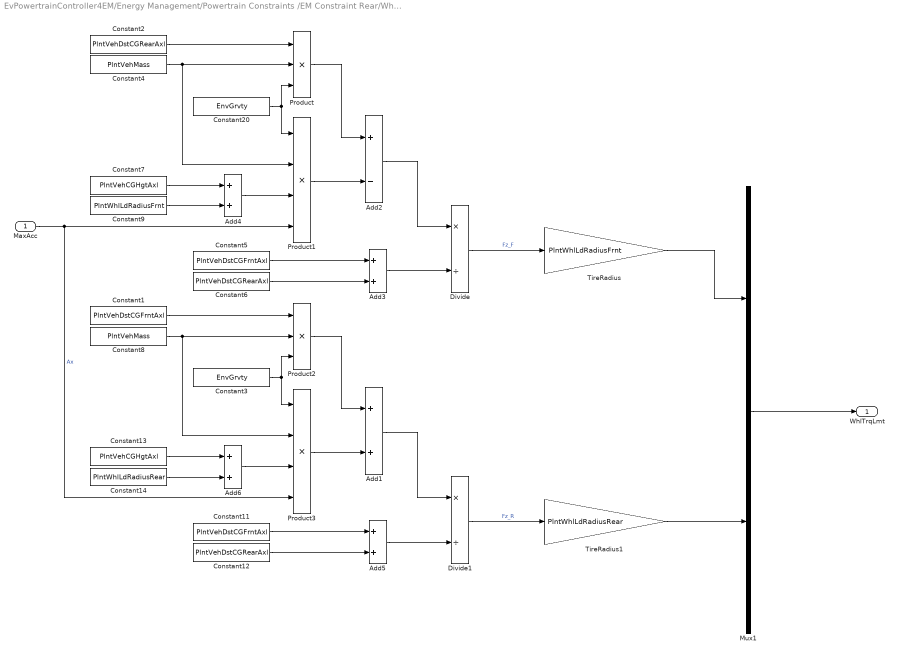
== system EvPowertrainController4EM/Energy Management/Powertrain Constraints /EM Constraint Rear/Wheel Torque Saturation for Max g Rates/Wheel Torque Limit at Max g Rates/Wheel Torque at Max Acceleration Rate ==
  MaxAcc : Inport
  Add{1,3..6} (5 alike) : Sum
  Add2 : Sum  Inputs=+-
  Constant1 : Constant  Value=PlntVehDstCGFrntAxl  SampleTime=-1
  Constant11 : Constant  Value=PlntVehDstCGFrntAxl  SampleTime=-1
  Constant12 : Constant  Value=PlntVehDstCGRearAxl  SampleTime=-1
  Constant13 : Constant  Value=PlntVehCGHgtAxl  SampleTime=-1
  Constant14 : Constant  Value=PlntWhlLdRadiusRear  SampleTime=-1
  Constant2 : Constant  Value=PlntVehDstCGRearAxl  SampleTime=-1
  Constant20 : Constant  Value=EnvGrvty  SampleTime=-1
  Constant3 : Constant  Value=EnvGrvty  SampleTime=-1
  Constant4 : Constant  Value=PlntVehMass  SampleTime=-1
  Constant5 : Constant  Value=PlntVehDstCGFrntAxl  SampleTime=-1
  Constant6 : Constant  Value=PlntVehDstCGRearAxl  SampleTime=-1
  Constant7 : Constant  Value=PlntVehCGHgtAxl  SampleTime=-1
  Constant8 : Constant  Value=PlntVehMass  SampleTime=-1
  Constant9 : Constant  Value=PlntWhlLdRadiusFrnt  SampleTime=-1
  Divide : Product  Inputs=*/
  Divide1 : Product  Inputs=*/
  Mux1 : Mux  Inputs=2
  Product : Product  Inputs=3
  Product1 : Product  Inputs=4
  Product2 : Product  Inputs=3
  Product3 : Product  Inputs=4
  TireRadius : Gain  Gain=PlntWhlLdRadiusFrnt
  TireRadius1 : Gain  Gain=PlntWhlLdRadiusRear
  WhlTrqLmt : Outport  VectorParamsAs1DForOutWhenUnconnected=off
  wires:
  Divide1/1 -> TireRadius1/1  "Fz_R"
  Product3/1 -> Add1/2
  Product2/1 -> Add1/1
  Constant11/1 -> Add5/1
  Constant8/1 -> Product3/2, Product2/2
  Add5/1 -> Divide1/2
  Add6/1 -> Product3/3
  Constant12/1 -> Add5/2
  Constant1/1 -> Product2/1
  Constant13/1 -> Add6/1
  Constant14/1 -> Add6/2
  Add1/1 -> Divide1/1
  Constant3/1 -> Product3/1, Product2/3
  Constant20/1 -> Product/3, Product1/1
  Mux1/1 -> WhlTrqLmt/1
  Add2/1 -> Divide/1
  Constant9/1 -> Add4/2
  Constant7/1 -> Add4/1
  Constant2/1 -> Product/1
  Constant6/1 -> Add3/2
  Divide/1 -> TireRadius/1  "Fz_F"
  Add4/1 -> Product1/3
  Add3/1 -> Divide/2
  MaxAcc/1 -> Product1/4, Product3/4  "Ax"
  Constant4/1 -> Product/2, Product1/2
  Constant5/1 -> Add3/1
  Product/1 -> Add2/1
  Product1/1 -> Add2/2
  TireRadius/1 -> Mux1/1
  TireRadius1/1 -> Mux1/2

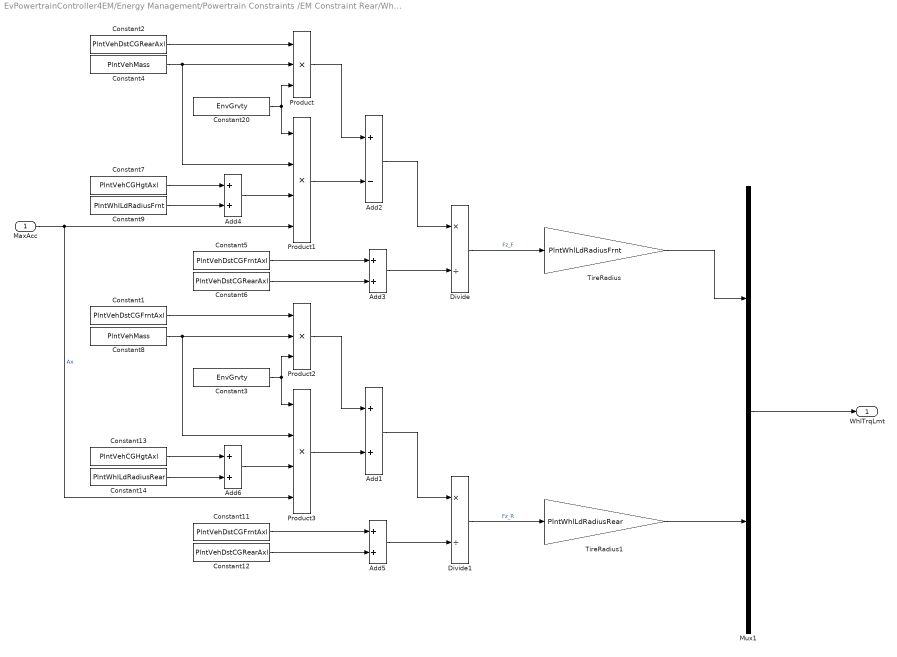
== system EvPowertrainController4EM/Energy Management/Powertrain Constraints /EM Constraint Rear/Wheel Torque Saturation for Max g Rates/Wheel Torque Limit at Max g Rates/Wheel Torque at Max Deceleration Rate ==
  MaxAcc : Inport
  Add{1,3..6} (5 alike) : Sum
  Add2 : Sum  Inputs=+-
  Constant1 : Constant  Value=PlntVehDstCGFrntAxl  SampleTime=-1
  Constant11 : Constant  Value=PlntVehDstCGFrntAxl  SampleTime=-1
  Constant12 : Constant  Value=PlntVehDstCGRearAxl  SampleTime=-1
  Constant13 : Constant  Value=PlntVehCGHgtAxl  SampleTime=-1
  Constant14 : Constant  Value=PlntWhlLdRadiusRear  SampleTime=-1
  Constant2 : Constant  Value=PlntVehDstCGRearAxl  SampleTime=-1
  Constant20 : Constant  Value=EnvGrvty  SampleTime=-1
  Constant3 : Constant  Value=EnvGrvty  SampleTime=-1
  Constant4 : Constant  Value=PlntVehMass  SampleTime=-1
  Constant5 : Constant  Value=PlntVehDstCGFrntAxl  SampleTime=-1
  Constant6 : Constant  Value=PlntVehDstCGRearAxl  SampleTime=-1
  Constant7 : Constant  Value=PlntVehCGHgtAxl  SampleTime=-1
  Constant8 : Constant  Value=PlntVehMass  SampleTime=-1
  Constant9 : Constant  Value=PlntWhlLdRadiusFrnt  SampleTime=-1
  Divide : Product  Inputs=*/
  Divide1 : Product  Inputs=*/
  Mux1 : Mux  Inputs=2
  Product : Product  Inputs=3
  Product1 : Product  Inputs=4
  Product2 : Product  Inputs=3
  Product3 : Product  Inputs=4
  TireRadius : Gain  Gain=PlntWhlLdRadiusFrnt
  TireRadius1 : Gain  Gain=PlntWhlLdRadiusRear
  WhlTrqLmt : Outport  VectorParamsAs1DForOutWhenUnconnected=off
  wires:
  TireRadius1/1 -> Mux1/2
  TireRadius/1 -> Mux1/1
  Product1/1 -> Add2/2
  Product/1 -> Add2/1
  Constant5/1 -> Add3/1
  Constant4/1 -> Product1/2, Product/2
  MaxAcc/1 -> Product3/4, Product1/4  "Ax"
  Add3/1 -> Divide/2
  Add4/1 -> Product1/3
  Divide/1 -> TireRadius/1  "Fz_F"
  Constant6/1 -> Add3/2
  Constant2/1 -> Product/1
  Constant7/1 -> Add4/1
  Constant9/1 -> Add4/2
  Add2/1 -> Divide/1
  Mux1/1 -> WhlTrqLmt/1
  Constant20/1 -> Product1/1, Product/3
  Constant3/1 -> Product2/3, Product3/1
  Add1/1 -> Divide1/1
  Constant14/1 -> Add6/2
  Constant13/1 -> Add6/1
  Constant1/1 -> Product2/1
  Constant12/1 -> Add5/2
  Add6/1 -> Product3/3
  Add5/1 -> Divide1/2
  Constant8/1 -> Product2/2, Product3/2
  Constant11/1 -> Add5/1
  Product2/1 -> Add1/1
  Product3/1 -> Add1/2
  Divide1/1 -> TireRadius1/1  "Fz_R"

== system EvPowertrainController4EM/Energy Management/Powertrain Constraints /EM Constraint Front/Tabular Power Loss Data/2EM or 3EM Dual Rear/WhlTrq2EMTrq/Diff Eta ==
  note: Pwr >= 0, v = 1
      | Pwr < 0, v= -1
  SpdIn : Inport
  TrqIn : Inport  Port=2
  Constant : Constant  Value=PlntDiffrntlEff*PlntEM1TransEff
  Constant1 : Constant  SampleTime=-1
  Constant2 : Constant  Value=-1  SampleTime=-1
  Math Function1 : Math  Operator=pow  SignedPower=on  OutputSignalType=real
  Product1 : Product
  Switch2 : Switch  SaturateOnIntegerOverflow=off  InputSameDT=off
  eta : Outport  VectorParamsAs1DForOutWhenUnconnected=off
  wires:
  SpdIn/1 -> Product1/2
  Constant/1 -> Math Function1/1
  Constant2/1 -> Switch2/3
  Constant1/1 -> Switch2/1
  Product1/1 -> Switch2/2
  Switch2/1 -> Math Function1/2
  Math Function1/1 -> eta/1
  TrqIn/1 -> Product1/1

== system EvPowertrainController4EM/Energy Management/Powertrain Constraints /EM Constraint Front/Tabular Power Loss Data/3EM Dual Front or 4EM/WhlTrq2EMTrq/Gear Eta ==
  SpdIn : Inport
  TrqIn : Inport  Port=2
  Constant : Constant  Value=PlntEMWhlGearEffFL*PlntEM1TransEff
  Constant1 : Constant  SampleTime=-1
  Constant2 : Constant  Value=-1  SampleTime=-1
  Math Function1 : Math  Operator=pow  SignedPower=on  OutputSignalType=real
  Product1 : Product
  Switch2 : Switch  SaturateOnIntegerOverflow=off  InputSameDT=off
  eta : Outport  VectorParamsAs1DForOutWhenUnconnected=off
  wires:
  TrqIn/1 -> Product1/1
  Math Function1/1 -> eta/1
  Switch2/1 -> Math Function1/2
  Product1/1 -> Switch2/2
  Constant1/1 -> Switch2/1
  Constant2/1 -> Switch2/3
  Constant/1 -> Math Function1/1
  SpdIn/1 -> Product1/2

== system EvPowertrainController4EM/Energy Management/Powertrain Constraints /EM Constraint Rear/Tabular Power Loss Data/2EM/WhlTrq2EMTrq/Diff Eta ==
  note: Pwr >= 0, v = 1
      | Pwr < 0, v= -1
  SpdIn : Inport
  TrqIn : Inport  Port=2
  Constant : Constant  Value=PlntDiffrntl2Eff*PlntEM2TransEff
  Constant1 : Constant  SampleTime=-1
  Constant2 : Constant  Value=-1  SampleTime=-1
  Math Function1 : Math  Operator=pow  SignedPower=on  OutputSignalType=real
  Product1 : Product
  Switch2 : Switch  SaturateOnIntegerOverflow=off  InputSameDT=off
  eta : Outport  VectorParamsAs1DForOutWhenUnconnected=off
  wires:
  SpdIn/1 -> Product1/2
  Constant/1 -> Math Function1/1
  Constant2/1 -> Switch2/3
  Constant1/1 -> Switch2/1
  Product1/1 -> Switch2/2
  Switch2/1 -> Math Function1/2
  Math Function1/1 -> eta/1
  TrqIn/1 -> Product1/1

== system EvPowertrainController4EM/Energy Management/Powertrain Constraints /EM Constraint Rear/Tabular Power Loss Data/3EM Dual Front/WhlTrq2EMTrq/Diff Eta ==
  note: Pwr >= 0, v = 1
      | Pwr < 0, v= -1
  SpdIn : Inport
  TrqIn : Inport  Port=2
  Constant : Constant  Value=PlntDiffrntl2Eff*PlntEM3TransEff
  Constant1 : Constant  SampleTime=-1
  Constant2 : Constant  Value=-1  SampleTime=-1
  Math Function1 : Math  Operator=pow  SignedPower=on  OutputSignalType=real
  Product1 : Product
  Switch2 : Switch  SaturateOnIntegerOverflow=off  InputSameDT=off
  eta : Outport  VectorParamsAs1DForOutWhenUnconnected=off
  wires:
  TrqIn/1 -> Product1/1
  Math Function1/1 -> eta/1
  Switch2/1 -> Math Function1/2
  Product1/1 -> Switch2/2
  Constant1/1 -> Switch2/1
  Constant2/1 -> Switch2/3
  Constant/1 -> Math Function1/1
  SpdIn/1 -> Product1/2

== system EvPowertrainController4EM/Energy Management/Powertrain Constraints /EM Constraint Rear/Tabular Power Loss Data/3EM Dual Rear or 4EM/WhlTrq2EMTrq/Gear Eta ==
  SpdIn : Inport
  TrqIn : Inport  Port=2
  Constant : Constant  Value=PlntEMWhlGearEffRL*PlntEM3TransEff
  Constant1 : Constant  SampleTime=-1
  Constant2 : Constant  Value=-1  SampleTime=-1
  Math Function1 : Math  Operator=pow  SignedPower=on  OutputSignalType=real
  Product1 : Product
  Switch2 : Switch  SaturateOnIntegerOverflow=off  InputSameDT=off
  eta : Outport  VectorParamsAs1DForOutWhenUnconnected=off
  wires:
  TrqIn/1 -> Product1/1
  Math Function1/1 -> eta/1
  Switch2/1 -> Math Function1/2
  Product1/1 -> Switch2/2
  Constant1/1 -> Switch2/1
  Constant2/1 -> Switch2/3
  Constant/1 -> Math Function1/1
  SpdIn/1 -> Product1/2

== matlab function EvPowertrainController4EM/Energy Management/Hamiltonian computation and minimization/MATLAB Function ==
  data: minH output; idx output; H input; InfFlag input; allInf output
function [minH, idx, allInf] = fcn(H, InfFlag)

if all(InfFlag) 
    [minH, idx] = min(H);
    allInf = 1;
else
    [minH, idx] = min(H);
    allInf = 0;
end

== matlab function EvPowertrainController4EM/Torque Vectoring/4EM/Torque Vectoring Split Function Front ==
  data: MaxTrq input; TrqLeftOut output; TrqLeft input; TrqRght input; TrqRghtOut output; TrqVec input; Enbl input; BrkThresh input; MinTrq input
function [TrqLeftOut, TrqRghtOut] = fcn(MaxTrq, TrqLeft, TrqRght, TrqVec, Enbl, BrkThresh, MinTrq)
% Enbl:= flag to turn on TV, true if steering wheel is turned and non-zero vehicle speed
% BrkThresh:= flag to turn on TV, true if not braking
TrqLmt = min(MaxTrq-abs(TrqLeft),MaxTrq-abs(TrqRght));
DeltaTrq = min(MinTrq, min(TrqLmt,abs(TrqVec)))*sign(TrqVec)*Enbl;% limit difference in torque between tires to +/-MinTrq and to max/min motor torque
if BrkThresh > 0 % Not braking. Use Torque vectoring
    TrqLeftOut = (TrqLeft+DeltaTrq);
    TrqRghtOut = (TrqRght-DeltaTrq);
else % ignore TV
    TrqLeftOut = TrqLeft;
    TrqRghtOut = TrqRght;
end

== matlab function EvPowertrainController4EM/Torque Vectoring/3EM/Torque Vectoring Split Function ==
  data: MaxTrq input; TrqLeftOut output; TrqLeft input; TrqRght input; TrqRghtOut output; TrqVec input; Enbl input; BrkThresh input; MinTrq input
function [TrqLeftOut, TrqRghtOut] = fcn(MaxTrq, TrqLeft, TrqRght, TrqVec, Enbl, BrkThresh, MinTrq)
% Enbl:= flag to turn on TV, true if steering wheel is turned and non-zero vehicle speed
% BrkThresh:= flag to turn on TV, true if not braking
TrqLmt = min(MaxTrq-abs(TrqLeft),MaxTrq-abs(TrqRght));
DeltaTrq = min(MinTrq, min(TrqLmt,abs(TrqVec)))*sign(TrqVec)*Enbl;% limit difference in torque between tires to +/-MinTrq and to max/min motor torque
if BrkThresh > 0 % Not braking. Use Torque vectoring
    TrqLeftOut = (TrqLeft+DeltaTrq);
    TrqRghtOut = (TrqRght-DeltaTrq);
else % ignore TV
    TrqLeftOut = TrqLeft;
    TrqRghtOut = TrqRght;
end

== matlab function EvPowertrainController4EM/Torque Vectoring/4EM/Torque Vectoring Split Function Rear ==
  data: MaxTrq input; TrqLeftOut output; TrqLeft input; TrqRght input; TrqRghtOut output; TrqVec input; Enbl input; BrkThresh input; MinTrq input
function [TrqLeftOut, TrqRghtOut] = fcn(MaxTrq, TrqLeft, TrqRght, TrqVec, Enbl, BrkThresh, MinTrq)
% Enbl:= flag to turn on TV, true if steering wheel is turned and non-zero vehicle speed
% BrkThresh:= flag to turn on TV, true if not braking
TrqLmt = min(MaxTrq-abs(TrqLeft),MaxTrq-abs(TrqRght));
DeltaTrq = min(MinTrq, min(TrqLmt,abs(TrqVec)))*sign(TrqVec)*Enbl;% limit difference in torque between tires to +/-MinTrq and to max/min motor torque
if BrkThresh > 0 % Not braking. Use Torque vectoring
    TrqLeftOut = (TrqLeft+DeltaTrq);
    TrqRghtOut = (TrqRght-DeltaTrq);
else % ignore TV
    TrqLeftOut = TrqLeft;
    TrqRghtOut = TrqRght;
end
